simulink model "FOQL_PDE_Solver_OutputFeedback"  (R2019a)
settings: Solver=VariableStepAuto  StartTime=0.0  StopTime=10  FixedStep=0.01  RelTol=1e-3
libraries: PDECharactLib x1, simulink x1
settings Model: Creator=kc5492  LastModifiedBy=User
settings SolverCC: ZeroCrossAlgorithm=Adaptive
settings DataIOCC: ReturnWorkspaceOutputs=off
settings DebuggingCC: PregeneratedLibrarySubsystemCodeDiagnostic=none  ArithmeticOperatorsInVariantConditions=warning
settings SFSimCC: SimUseLocalCustomCode=off
settings RTWCC: RTWUseLocalCustomCode=off

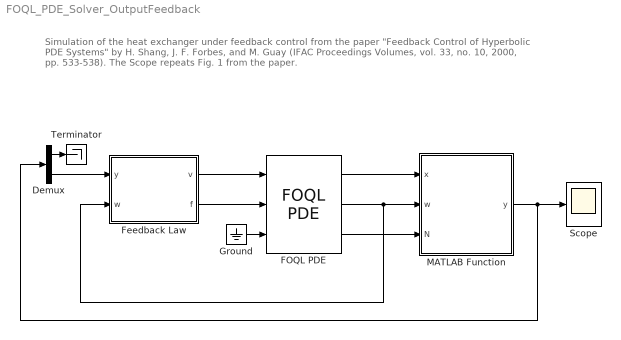
== system FOQL_PDE_Solver_OutputFeedback ==
  note: Simulation of the heat exchanger under feedback control from the paper "Feedback Control of Hyperbolic PDE Systems"
      | by H. Shang, J. F. Forbes, and M. Guay (IFAC Proceedings Volumes, vol. 33, no. 10, 2000, pp. 533-538).
      |
      | The Scope repeats Fig. 1 from the paper.
  Demux : Demux  Outputs=[3 1]
  FOQL PDE : PDECharactLib/FOQL PDE  ell=1  Nmax=100  x0=0:0.1:1  w0=1 - exp(-5.*(0:0.1:1))  initX=0  initW=0  dx=0.1  dw=0.1  dt=0.1  crossing_tol=1e-11  overflow_err=off
  Feedback Law : Subsystem  mask{k_1=5/3, alpha=1, T_j=10, k_2=5, tau_I=2, y_d=3}
      mask help: The initialization parameters v_I0 and y_0 can be adapted using the "Initialization" flag of the Mask Editor.
      mask init:
      | y_0 = 1-exp(-5);
      | v_I0 = tau_I*(y_d-y_0+alpha/k_2*(y_0-T_j));
  Ground : Ground
  MATLAB Function : MATLAB Function  TreatAsAtomicUnit=on
  Scope : Scope
  Terminator : Terminator
  wires:
  Feedback Law/1(v) -> FOQL PDE/1
  Feedback Law/2(f) -> FOQL PDE/2
  FOQL PDE/1 -> MATLAB Function/1(x)
  FOQL PDE/2 -> Feedback Law/2(w), MATLAB Function/2(w)
  FOQL PDE/3 -> MATLAB Function/3(N)
  MATLAB Function/1(y) -> Scope/1, Demux/1
  Demux/1 -> Terminator/1
  Demux/2 -> Feedback Law/1(y)
  Ground/1 -> FOQL PDE/3

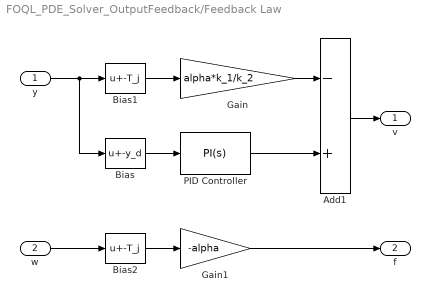
== system FOQL_PDE_Solver_OutputFeedback/Feedback Law ==
  y : Inport
  w : Inport  Port=2
  Add1 : Sum  Inputs=-+
  Bias : Bias  Bias=-y_d
  Bias1 : Bias  Bias=-T_j
  Bias2 : Bias  Bias=-T_j
  Gain : Gain  Gain=alpha*k_1/k_2
  Gain1 : Gain  Gain=-alpha
  PID Controller : simulink/Continuous/PID Controller  Controller=PI  Form=Parallel  TimeDomain=Continuous-time  SampleTime=-1  IntegratorMethod=Forward Euler  FilterMethod=Forward Euler  ControllerParametersSource=internal  P=k_1  I=k_1/tau_I  D=0  UseFilter=on  N=100  TunerSelectOption=Transfer Function Based (PID Tuner App)  InitialConditionSource=internal  InitialConditionForIntegrator=v_I0  InitialConditionForFilter=0  DifferentiatorICPrevScaledInput=0  ExternalReset=none  TrackingMode=off  Kt=1  LimitOutput=off  UpperSaturationLimit=inf  LowerSaturationLimit=-inf  LinearizeAsGain=on  AntiWindupMode=none  Kb=1  POutMin=[]  POutMax=[]  IOutMin=[]  IOutMax=[]  DOutMin=[]  DOutMax=[]  NOutMin=[]  NOutMax=[]  SumOutMin=[]  SumOutMax=[]  SaturationOutMin=[]  SaturationOutMax=[]  PParamMin=[]  PParamMax=[]  IParamMin=[]  IParamMax=[]  DParamMin=[]  DParamMax=[]  NParamMin=[]  NParamMax=[]  KbParamMin=[]  KbParamMax=[]  KtParamMin=[]  KtParamMax=[]  KbOutMin=[]  KbOutMax=[]  KtOutMin=[]  KtOutMax=[]  IntegratorOutMin=[]  IntegratorOutMax=[]  FilterOutMin=[]  FilterOutMax=[]  SumI1OutMin=[]  SumI1OutMax=[]  SumI2OutMin=[]  SumI2OutMax=[]  SumI3OutMin=[]  SumI3OutMax=[]  SumI4OutMin=[]  SumI4OutMax=[]  SumDOutMin=[]  SumDOutMax=[]  DifferentiatorOutMin=[]  DifferentiatorOutMax=[]  FilterDiffOutCoefMin=[]  FilterDiffOutCoefMax=[]  ReciprocalOutMin=[]  ReciprocalOutMax=[]  SumDenOutMin=[]  SumDenOutMax=[]  SumNumOutMin=[]  SumNumOutMax=[]  DivideOutMin=[]  DivideOutMax=[]  IntegratorContinuousStateAttributes=''  IntegratorStateMustResolveToSignalObject=off  IntegratorRTWStateStorageClass=Auto  FilterContinuousStateAttributes=''  FilterStateMustResolveToSignalObject=off  FilterRTWStateStorageClass=Auto  ParallelPVariant=InternalParameters  IdealPVariant=Disabled  IVariant=InternalParameters  DVariant=Disabled  IntegratorVariant=Continuous  SatVariant=Disabled  AWVariant=Passthrough  PCopyVariant=Disabled  TRVariant=Disabled  FdbkBlocksVariant=Forward  IdealPFdbkVariant=Disabled  SatFdbkVariant=Disabled  DerivativeFilterVariant=Disabled  NVariant=Disabled  NCopyVariant=Disabled_SignalSpec  FilterICVariant=Disabled  IntegratorICVariant=InternalICs  ExternalResetVariant=Disabled  TRSumVariant=Passthrough  SumFdbkVariant=Disabled  SumVariant=Sum_PI
  v : Outport
  f : Outport  Port=2
  wires:
  Bias2/1 -> Gain1/1
  Add1/1 -> v/1
  PID Controller/1 -> Add1/2
  Bias1/1 -> Gain/1
  y/1 -> Bias/1, Bias1/1
  w/1 -> Bias2/1
  Bias/1 -> PID Controller/1
  Gain1/1 -> f/1
  Gain/1 -> Add1/1

== matlab function FOQL_PDE_Solver_OutputFeedback/MATLAB Function ==
  data: x input; y output; w input; N input
function y = output(x, w, N)

y = interp1(x(1:N), w(1:N), [0.2, 0.5, 0.8, 1]);
